simulink library "move_index_lib"  (R2020b)
settings: Solver=VariableStepAuto  StartTime=0.0  StopTime=10.0  RelTol=1e-3
values from neighbouring files (symbols this model uses):
  kRollOverAdjustment = int16(1)    [move_index_params.m]
undefined symbols (not defined in the file or in its folder): kContainerLength, kFirstContainerIndex, kLastContainerIndex
libraries: simulink x1
settings Model: Creator=rsub  LastModifiedBy=rsub

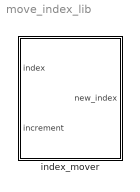
== system move_index_lib ==
  index_mover : Subsystem

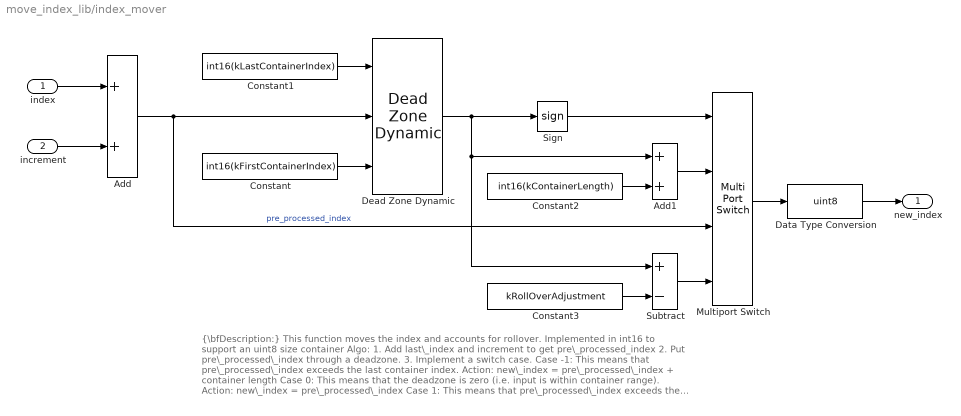
== system move_index_lib/index_mover ==
  note: {\bfDescription:}
      | This function moves the index and accounts for rollover. Implemented in int16 to support an uint8 size container
      |
      | Algo:
      | 1. Add last\_index and increment to get pre\_processed_index
      | 2. Put pre\_processed\_index through a deadzone.
      | 3. Implement a switch case.
      | Case -1:
      | This means that pre\_processed\_index exceeds the last container index. Action: new\_index = pre\_processed\_index + container length
      | Case 0:
      | This means that the deadzone is zero (i.e. input is within container range). Action: new\_index = pre\_processed\_index
      | Case 1:
      | This means that pre\_processed\_index exceeds the first container index. Action: new\_index = pre\_processed\_index - 1
      |
      | 4. Cast output back to uint8
  index : Inport
  increment : Inport  Port=2
  Add : Sum  OutDataTypeStr=int16
  Add1 : Sum
  Constant : Constant  Value=int16(kFirstContainerIndex)
  Constant1 : Constant  Value=int16(kLastContainerIndex)
  Constant2 : Constant  Value=int16(kContainerLength)
  Constant3 : Constant  Value=kRollOverAdjustment
  Data Type Conversion : DataTypeConversion  OutDataTypeStr=uint8
  Dead Zone Dynamic : simulink/Discontinuities/Dead Zone Dynamic
      settings: SourceProductBaseCode=SL
  Multiport Switch : MultiPortSwitch  DataPortOrder=Specify indices  DataPortIndices={-1,0,1}
  Sign : Signum
  Subtract : Sum  Inputs=+-
  new_index : Outport
  wires:
  Data Type Conversion/1 -> new_index/1
  Multiport Switch/1 -> Data Type Conversion/1
  Constant1/1 -> Dead Zone Dynamic/1
  index/1 -> Add/1
  Add/1 -> Dead Zone Dynamic/2, Multiport Switch/3  "pre_processed_index"
  Dead Zone Dynamic/1 -> Add1/1, Subtract/1, Sign/1
  Constant2/1 -> Add1/2
  Sign/1 -> Multiport Switch/1
  increment/1 -> Add/2
  Add1/1 -> Multiport Switch/2
  Constant/1 -> Dead Zone Dynamic/3
  Subtract/1 -> Multiport Switch/4
  Constant3/1 -> Subtract/2
